simulink model "RobustCAD_Model"  (R2025b)
settings: Solver=VariableStepAuto  StartTime=0.0  StopTime=10.0  RelTol=1e-3
settings Model: Creator=tudor  LastModifiedBy=tudor

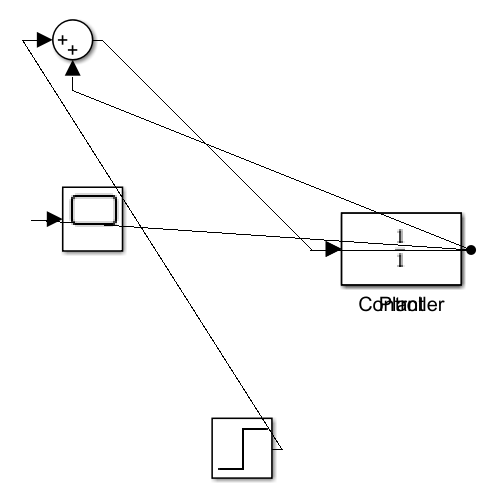
[thumbnail: Simulink's stored preview of the top-level diagram]
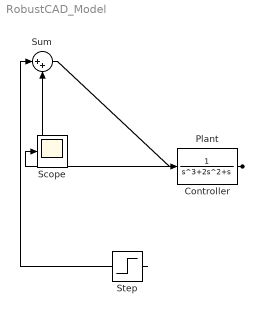
== system RobustCAD_Model ==
  Controller : TransferFcn  Denominator=[1]
  Plant : TransferFcn  Numerator=[0 0 0 1]  Denominator=[1 2 1 0]
  Scope : Scope
  Step : Step  SampleTime=0
  Sum : Sum  Inputs=|++
  wires:
  Step/1 -> Sum/1
  Sum/1 -> Controller/1
  Controller/1 -> Plant/1
  Plant/1 -> Scope/1, Sum/2
